simulink model "mpc_winter1"  (R2017b)
settings: Solver=VariableStepAuto  StartTime=0.0  StopTime=86400  RelTol=1e-3
model workspace: external: MAT-File /home/wcl-lab/Desktop/FromAryan-PC/matlab_winter.mat (data not in the file)
values from neighbouring files (symbols this model uses):
  Ts = 1800    [matlab_summer.mat]    (also in matlab_winter.mat; transferfunc_summer.m; transferfunc_winter.m)
libraries: mpclib x1, realtime_pacer_lib x1, dspsrcs4 x1
settings Model: Creator=root  LastModifiedBy=root
settings DataIOCC: OutputSaveName=u
settings DebuggingCC: AlgebraicLoopMsg=none  ArtificialAlgebraicLoopMsg=none
settings HardwareCC: ProdBitPerLong=64  ProdHWDeviceType=Intel->x86-64 (Linux 64)

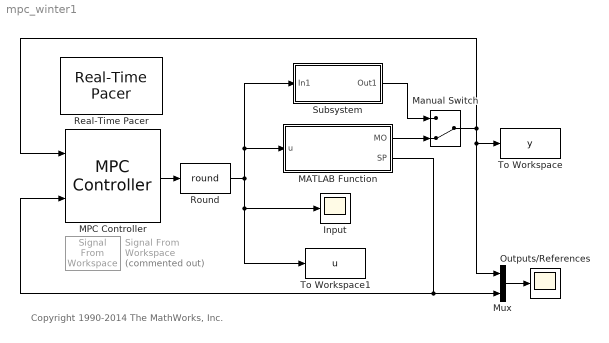
== system mpc_winter1 ==
  note: Copyright 1990-2014 The MathWorks, Inc.
  Input : Scope
  MATLAB Function : MATLAB Function  TreatAsAtomicUnit=on
  MPC Controller : mpclib/MPC Controller  mpcobj=mpcobj  is_multiple=0  enable_value=0  return_u0=off  ref_from_ws=off  ref_signal_name=[]  ref_preview=on  md_from_ws=off  md_signal_name=[]  md_preview=on  from_project=off  project_file=MPCtask.mat  md_inport=off  mv_inport=off  cost_outport=off  return_sequence=off  return_qpstatus=off  return_state=off  state_inport=off  lims_inport=off  cc_inport=off  ywt_inport=off  is_designfromscratch=0  uwt_inport=off  duwt_inport=off  rhoeps_inport=off  uref_inport=off  n_ts=1800  n_p=48  n_mv=1  n_md=0  n_ud=0  n_mo=1  n_uo=0  BlockDataType=double  SampleTimeInherited=off  switch_inport=off
  Manual Switch : ManualSwitch  CurrentSetting=0
  Mux : Mux  Inputs=2
  Outputs/References : Scope
  Real-Time Pacer : realtime_pacer_lib/Real-Time Pacer  simTimePerRealTime=1
  Round : Rounding  Operator=round
  Signal From Workspace : dspsrcs4/Signal From Workspace  Commented=on  X=setpoint  Ts=Ts  nsamps=1  OutputAfterFinalValue=Cyclic repetition  ignoreOrWarnInputAndFrameLengths=off  OutputFrames=off
  Subsystem : Subsystem  TreatAsAtomicUnit=on
      settings: MinAlgLoopOccurrences=on
  To Workspace : ToWorkspace  VariableName=y  SampleTime=Ts
      settings: MaxDataPoints=Inf
  To Workspace1 : ToWorkspace  VariableName=u  SampleTime=-1
      settings: MaxDataPoints=Inf
  wires:
  MATLAB Function/1(MO) -> Manual Switch/2
  MPC Controller/1 -> Round/1
  Subsystem/1(Out1) -> Manual Switch/1
  Round/1 -> Input/1, To Workspace1/1, Subsystem/1(In1), MATLAB Function/1(u)
  Manual Switch/1 -> To Workspace/1, Mux/1, MPC Controller/1
  Mux/1 -> Outputs/References/1
  MATLAB Function/2(SP) -> MPC Controller/2, Mux/2

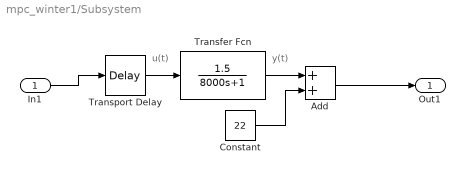
== system mpc_winter1/Subsystem ==
  note: u(t)
  note: y(t)
  In1 : Inport
  Add : Sum
  Constant : Constant  Value=22  SampleTime=1
  Transfer Fcn : TransferFcn  Numerator=[1.5]  Denominator=[8000 1]
  Transport Delay : TransportDelay  DelayTime=700
  Out1 : Outport
  wires:
  In1/1 -> Transport Delay/1
  Transport Delay/1 -> Transfer Fcn/1
  Add/1 -> Out1/1
  Constant/1 -> Add/2
  Transfer Fcn/1 -> Add/1

== matlab function mpc_winter1/MATLAB Function ==
  settings: sampleTime=Ts
  data: u input; MO output; SP output
function [MO,SP] = fcn(u)
    coder.extrinsic('fscanf');
    fid1 = fopen('/home/wcl-lab/input','w');
    fid2 = fopen('/home/wcl-lab/measured_output','r');
    fid3 = fopen('/home/wcl-lab/setpoint','r');
    t1 = fscanf(fid3,'%f');
    SP = zeros(1,1);
    SP = t1;
    t = fscanf(fid2,'%f');
    MO = zeros(1,1);
    MO = t;
    if u==1   
        fprintf(fid1,int2str(1));
        fprintf(fid1,'\n');
    end
    if u==0   
        fprintf(fid1,int2str(0));
        fprintf(fid1,'\n');
    end
    fclose(fid1);
    fclose(fid2);
    fclose(fid3);
end
